simulink model "Ex312"  (R2021b)
settings: Solver=VariableStepAuto  StartTime=0.0  StopTime=10.0  RelTol=1e-3
settings Model: Creator=abdul  LastModifiedBy=abdul

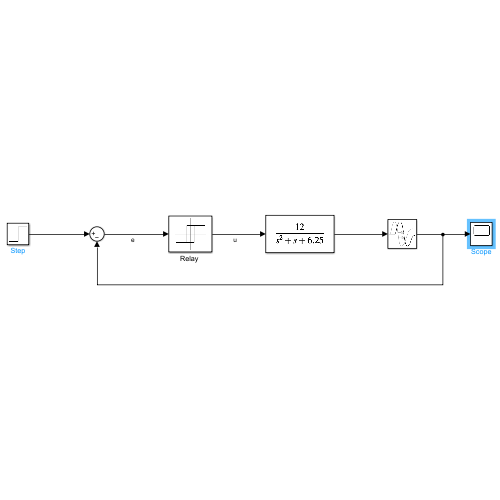
[thumbnail: Simulink's stored preview of the top-level diagram]
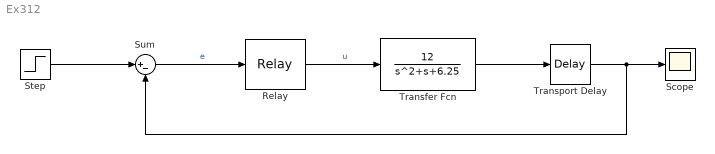
== system Ex312 ==
  "Relay " : Relay  OnSwitchValue=1  OffSwitchValue=-1  OnOutputValue=2  OffOutputValue=-2
  Scope : Scope
  Step : Step  Time=10  SampleTime=0
  Sum : Sum  Inputs=|+-
  Transfer Fcn : TransferFcn  Numerator=[12]  Denominator=[1 1 6.25]
  Transport Delay : TransportDelay  DelayTime=5
  wires:
  "Relay "/1 -> Transfer Fcn/1  "u"
  Sum/1 -> "Relay "/1  "e"
  Step/1 -> Sum/1
  Transfer Fcn/1 -> Transport Delay/1
  Transport Delay/1 -> Scope/1, Sum/2
